simulink model "ExperimentalCarrier_longitudinal"  (R2015b)
settings: Solver=ode45  StartTime=0.0  StopTime=60  FixedStep=0.001  RelTol=1e-4
model workspace (MAT data in the model file):
  CX = [-0.020017155432; -0.0250180932111; -0.030544767781; -0.0366030177792; -0.0431954569041]
  CX_P = [-3.8788104025e-05; -0.000157009586721; -8.33005923499e-05; 4.36263205191e-05; 8.75463477638e-05]
  CX_Q = [-0.207993391526; -0.236116645752; -0.264091029583; -0.292079605385; -0.320346819683]
  CX_R = [0.00103448390012; 0.00120711118767; 0.00133502371584; 0.00146905219193; 0.0016515166303]
  CX_d = reshape([-0.0179596722301 -0.0197556406443 -0.0215296927775 -0.0233172355081 -0.0251411734088 0.00353274771863 0.00408472673345 0.00460460396215 0.00513024749002 0.00568462730478], [5 1 2])
  CX_d_elevator = [-0.0179596722301; -0.0197556406443; -0.0215296927775; -0.0233172355081; -0.0251411734088]
  CX_d_rudder = [0.00353274771863; 0.00408472673345; 0.00460460396215; 0.00513024749002; 0.00568462730478]
  CY = [-4.5217922426e-06; 5.22435851707e-05; 0.000183887113454; 0.000333475068731; 0.000452221434108]
  CY_P = [0.352257019544; 0.363263703068; 0.372310862359; 0.376200975649; 0.377300019734]
  CY_Q = [0.110043766373; 0.11079927373; 0.112561154643; 0.114510099317; 0.116086067683]
  CY_R = [-0.326040929997; -0.32773612119; -0.329287944874; -0.33055019267; -0.331668414023]
  CY_d = reshape([0.0148975523026 0.0150362935124 0.015237582339 0.0154527280836 0.0156448316098 -0.13717454765 -0.137491342129 -0.137816916372 -0.138147259306 -0.138463716116], [5 1 2])
  CY_d_elevator = [0.0148975523026; 0.0150362935124; 0.015237582339; 0.0154527280836; 0.0156448316098]
  CY_d_rudder = [-0.13717454765; -0.137491342129; -0.137816916372; -0.138147259306; -0.138463716116]
  CZ = [0.433918417301; 0.474298454266; 0.514671186482; 0.555148813041; 0.595722799276]
  CZ_P = [0.00129613826783; 0.00442759554205; 0.00267513559452; 0.000223228043457; -0.00031135300856]
  CZ_Q = [7.41020869928; 7.41837707941; 7.42599317709; 7.43441633219; 7.4434283008]
  CZ_R = [-0.030484458254; -0.0314562905176; -0.0323752658756; -0.0334837032738; -0.0349135867002]
  CZ_d = reshape([0.557451970659 0.557751465503 0.557962985265 0.558156625973 0.558318687373 -0.104459514841 -0.104809350426 -0.105143668837 -0.105483709566 -0.105819316132], [5 1 2])
  CZ_d_elevator = [0.557451970659; 0.557751465503; 0.557962985265; 0.558156625973; 0.558318687373]
  CZ_d_rudder = [-0.104459514841; -0.104809350426; -0.105143668837; -0.105483709566; -0.105819316132]
  Cl = [-1.35607961429e-06; -5.96188071166e-06; -1.67033646109e-05; -2.94231268293e-05; -4.01077970867e-05]
  Cl_P = [-0.439205034752; -0.440723709414; -0.442152638591; -0.443068299499; -0.443627112534]
  Cl_Q = [-0.00917034469699; -0.00927738512973; -0.00949166137223; -0.00975372945302; -0.0100173762744]
  Cl_R = [0.0707908045152; 0.0708836498468; 0.0709529443546; 0.0709782004888; 0.0709702581948]
  Cl_d = reshape([-0.00125631208593 -0.00127240477427 -0.00129594809443 -0.00132394457069 -0.00135365672185 0.0120340930302 0.0120431420253 0.0120538349209 0.012065931941 0.0120777084325], [5 1 2])
  Cl_d_elevator = [-0.00125631208593; -0.00127240477427; -0.00129594809443; -0.00132394457069; -0.00135365672185]
  Cl_d_rudder = [0.0120340930302; 0.0120431420253; 0.0120538349209; 0.012065931941; 0.0120777084325]
  Cm = [0.0125955960448; 0.00755459695358; 0.00246646731807; -0.00292807143153; -0.00862510234146]
  Cm_P = [-0.00284218408989; -0.0097092504066; -0.00585776139249; -0.000486652887433; 0.000677869990232]
  Cm_Q = [-9.33029736541; -9.33733537595; -9.34332688954; -9.35122395193; -9.36051345323]
  Cm_R = [0.0662348186498; 0.0683959531597; 0.0704584936088; 0.0729594772358; 0.0761904930638]
  Cm_d = reshape([-1.26929427701 -1.2696185084 -1.26973590838 -1.26980240453 -1.26978468603 0.228767161047 0.229455531687 0.230105888147 0.230769688943 0.231425434534], [5 1 2])
  Cm_d_elevator = [-1.26929427701; -1.2696185084; -1.26973590838; -1.26980240453; -1.26978468603]
  Cm_d_rudder = [0.228767161047; 0.229455531687; 0.230105888147; 0.230769688943; 0.231425434534]
  Cn = [-2.39196708194e-06; 2.19531005211e-05; 7.80516594694e-05; 0.000141460168108; 0.000191546816275]
  Cn_P = [-0.0138852805825; -0.0104525390167; -0.00804029890533; -0.00770122144879; -0.00830785414203]
  Cn_Q = [0.0468266728784; 0.0471357484906; 0.0478735856255; 0.0486865128781; 0.0493357339708]
  Cn_R = [-0.112685214148; -0.113184603314; -0.113623636715; -0.113957068484; -0.114242510185]
  Cn_d = reshape([0.00634316820633 0.00640010611535 0.00648337961591 0.00657205165139 0.00665055318483 -0.0584904156504 -0.058612540103 -0.0587418941859 -0.0588730038419 -0.0589956355318], [5 1 2])
  Cn_d_elevator = [0.00634316820633; 0.00640010611535; 0.00648337961591; 0.00657205165139; 0.00665055318483]
  Cn_d_rudder = [-0.0584904156504; -0.058612540103; -0.0587418941859; -0.0588730038419; -0.0589956355318]
  InertiaTensor = [1  0  0; 0  1  0; 0  0  1]
  alpha = [0.0698131700798; 0.0785398163397; 0.0872664625997; 0.0959931088597; 0.10471975512]
  alpha_ini = 0
  beta = 0
  centerOfGravity = -0.092
  estimatedVelocity = 14
  mass = 1.56
  mean_chord = 0.25
  q_ini = 0
  spanwidth = 1.5
  theta_ini = 0
undefined symbols (not defined in the file): Earth, m, s, U0, w0, WGS84
libraries: aerolibconvert2 x6, aerolibasang x2, aerolibfltsims x2, aerolib3dof2 x1, aerolibadyn x1, aerolibtransform2 x1, aerolibanimutils x1, aerolibatmos2 x1, aerolibgravity2 x1
settings Model: Creator=jruesch  LastModifiedBy=jruesch
settings DataIOCC: SaveFormat=Array
settings OptimizationCC: BlockReduction=off
settings HardwareCC: ProdBitPerPointer=32  ProdLargestAtomicFloat=None  ProdIntDivRoundTo=Undefined  ProdEndianess=Unspecified  ProdWordSize=32  ProdHWDeviceType=32-bit Generic
settings GRTTargetCC: GeneratePreprocessorConditionals=Disable all
settings ConfigComp: CovModelRefEnable=Off

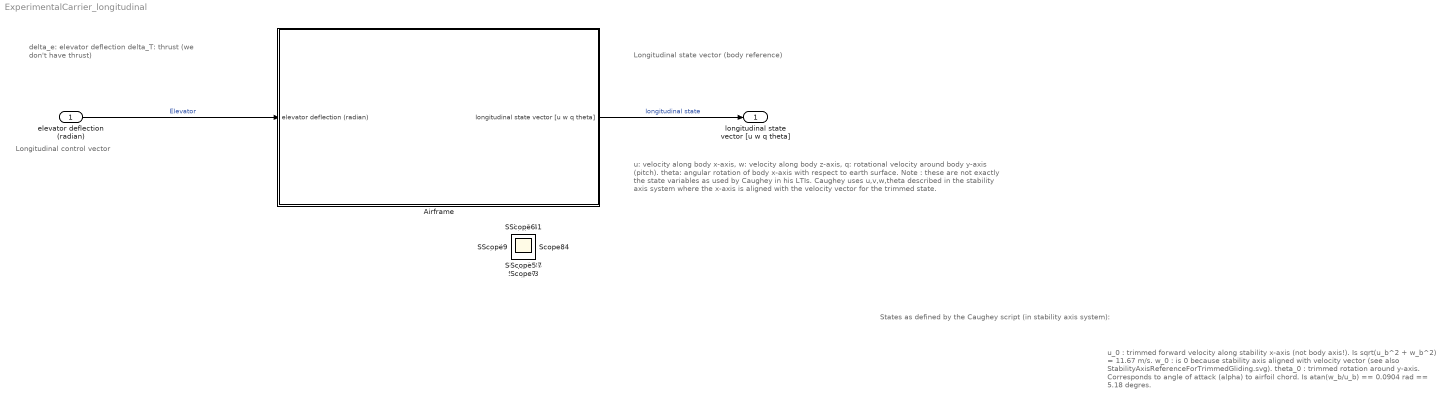
== system ExperimentalCarrier_longitudinal ==
  note: States as defined by the Caughey script (in stability axis system):
  note: u_0 : trimmed forward velocity along stability x-axis (not body axis!).
      | Is sqrt(u_b^2 + w_b^2) = 11.67 m/s.
      | w_0 : is 0 because stability axis aligned with velocity vector
      | (see also StabilityAxisReferenceForTrimmedGliding.svg).
      | theta_0 : trimmed rotation around y-axis. Corresponds
      | to angle of attack (alpha) to airfoil chord.
      | Is atan(w_b/u_b) == 0.0904 rad == 5.18 degres.
  note: delta_e: elevator deflection
      | delta_T: thrust (we don't have thrust)
  note: Longitudinal control vector
  note: u: velocity along body x-axis,
      | w: velocity along body z-axis,
      | q: rotational velocity around body y-axis (pitch).
      | theta: angular rotation of body x-axis with respect to earth surface.
      |
      | Note : these are not exactly the state variables as used by Caughey in his LTIs.
      | Caughey uses u,v,w,theta described in the stability axis system where the x-axis is aligned
      | with the velocity vector for the trimmed state.
  note: Longitudinal state vector (body reference)
  elevator deflection (radian) : Inport
  Airframe : Subsystem
      mask Display: image(imread('../../figures/Airframe.png'))
  longitudinal state vector [u w q theta] : Outport
  Scope{,1..41,43..45} (45 alike) : Scope
  wires:
  elevator deflection (radian)/1 -> Airframe/1(elevator deflection (radian))  "Elevator"
  Airframe/1(longitudinal state vector [u w q theta]) -> longitudinal state vector [u w q theta]/1  "longitudinal state"

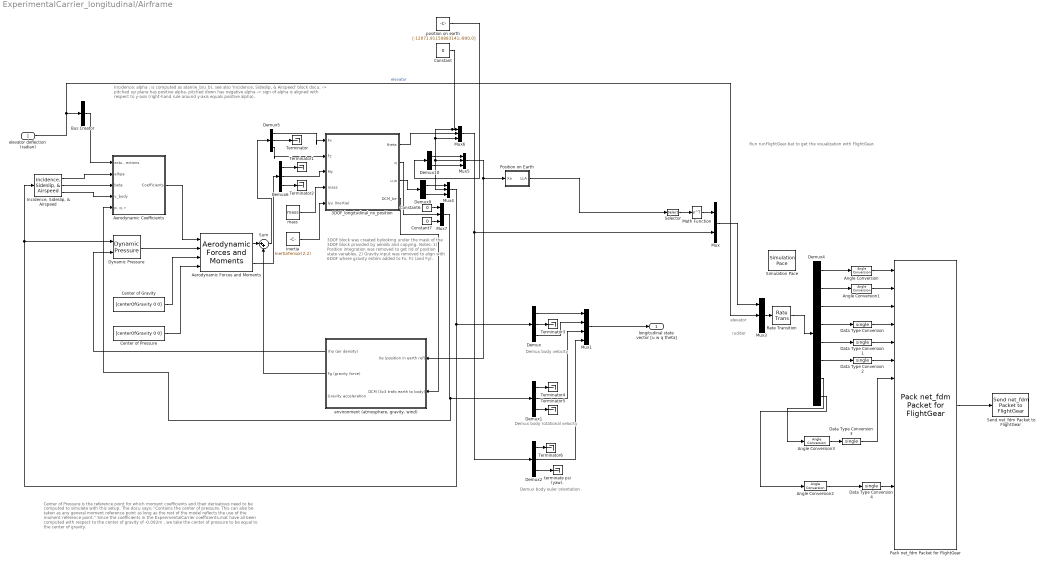
== system ExperimentalCarrier_longitudinal/Airframe ==
  note: 3DOF block was created bylooking under the mask of the 3DOF block provided by aerolib and copying.
      |
      | Notes:
      | 1) Position integration was removed to get rid of position state variables.
      | 2) Gravity input was removed to align with 6DOF where
      | gravity enters added to Fx, Fz (and Fy).
  note: rudder
  note: elevator
  note: Incidence:
      | alpha : is computed as atan(w_b/u_b), see also 'Incidence, Sideslip, & Airspeed' block docu.
      | -> pitched up plane has positive alpha, pitched down has negative alpha
      | -> sign of alpha is aligned with respect to y-axis (right-hand rule around y-axis equals positive alpha).
  note: Demux body velocity
  note: Run runFlightGear.bat to get the visualization with FlightGear.
  note: Center of Pressure is the reference point for which moment coefficients and their derivatives need to be computed to simulate with this setup.
      | The docu says: "Contains the center of pressure. This can also be taken as any general moment reference point as long as the rest of the model reflects the use of the moment reference point." Since the coefficients in the ExperimentalCarrier coefficients.mat have all been computed with respect to the center of gravity of -0.092m , we take the center of pressure to be equal to the center of gravity.
  note: Demux body rotational velocity
  note: Demux body euler orientation
  elevator deflection (radian) : Inport
  3DOF_longitudinal_no_position : Subsystem
  "Aerodynamic Forces and Moments " : aerolibadyn/Aerodynamic Forces and Moments   inputAxes=Body  outputForceAxes=Body  outputMomentAxes=Body  S=spanwidth*mean_chord  b=spanwidth  cbar=mean_chord
  Aerodynamic Coefficients : Subsystem
  Angle Conversion : aerolibconvert2/Angle Conversion  IU=deg  OU=rad
  Angle Conversion1 : aerolibconvert2/Angle Conversion  IU=deg  OU=rad
  Angle Conversion2 : aerolibconvert2/Angle Conversion  IU=rad  OU=deg
  Angle Conversion3 : aerolibconvert2/Angle Conversion  IU=rad  OU=deg
  Bus Creator : BusCreator  Inputs=1
  Center of Gravity : Constant  Value=[centerOfGravity 0 0]
  Center of Pressure : Constant  Value=[centerOfGravity 0 0]
  Constant : Constant  Value=0
  Constant6 : Constant  Value=0
  Constant7 : Constant  Value=0
  Data Type Conversion{,1..4} (5 alike) : DataTypeConversion  OutDataTypeStr=single
  Demux{,1..2,5..6} (5 alike) : Demux  Outputs=3
  Demux10 : Demux  Outputs=2
  Demux4 : Demux  Outputs=8
  Demux9 : Demux  Outputs=2
  Dynamic Pressure : aerolibasang/Dynamic Pressure
  "Incidence, Sideslip, & Airspeed" : aerolibasang/Incidence, Sideslip, & Airspeed
  Inertia : Constant  Value=InertiaTensor(2,2)
  Math Function : Math  Operator=transpose  SaturateOnIntegerOverflow=on
  Mux : Mux  Inputs=2
  Mux1 : Mux
  Mux{3..7} (5 alike) : Mux  Inputs=3
  Pack net_fdm Packet for FlightGear : aerolibfltsims/Pack net_fdm Packet for FlightGear  FlightGearVersion=v3.4  ShowPositionAttitudeInputs=on  ShowVelocityAccelerationInputs=off  ShowControlSurfacePositionInputs=on  ShowEngineFuelInputs=off  ShowLandingGearInputs=off  ShowEnvironmentInputs=off  SampleTime=1/30
  Position on Earth : Subsystem  Priority=1  TreatAsAtomicUnit=on
  Rate Transition : RateTransition  Integrity=off  OutPortSampleTime=1/30
  Selector : Selector  InputPortWidth=3  IndexOptions=Index vector (dialog)  Indices=[2 1 3]  OutputSizes=1
  Send net_fdm Packet to FlightGear : aerolibfltsims/Send net_fdm Packet to FlightGear  DestinationIpAddress=127.0.0.1  DestinationPort=5502  LocalIpPort=-1  varLen=off  SampleTime=1/30
  Simulation Pace : aerolibanimutils/Simulation Pace  SimulationPace=1  SleepMode=MATLAB Thread  OutputPaceError=off  SampleTime=1/30
      settings: AttributesFormatString=%<SimulationPace> sec/sec
  Sum : Sum  Inputs=|++
  Terminator{,1..6} (7 alike) : Terminator
  "environment (atmosphere, gravity, wind)" : Subsystem
  mass : Constant  Value=mass
  position on earth : Constant  Value=[-12071.91150883141;-800.0]
  terminate psi (yaw). : Terminator
  longitudinal state vector [u w q theta] : Outport
  wires:
  "Aerodynamic Forces and Moments "/1 -> Sum/1
  "Aerodynamic Forces and Moments "/2 -> Demux6/1
  Center of Gravity/1 -> "Aerodynamic Forces and Moments "/3
  Center of Pressure/1 -> "Aerodynamic Forces and Moments "/4
  Dynamic Pressure/1 -> "Aerodynamic Forces and Moments "/2
  Position on Earth/1(LLA) -> Selector/1
  Math Function/1 -> Mux/1
  Mux/1 -> Mux3/1
  Selector/1 -> Math Function/1
  "environment (atmosphere, gravity, wind)"/1(rho (air density)) -> Dynamic Pressure/2
  "Incidence, Sideslip, & Airspeed"/1 -> Aerodynamic Coefficients/2(alhpa)
  "Incidence, Sideslip, & Airspeed"/2 -> Aerodynamic Coefficients/3(beta)
  "Incidence, Sideslip, & Airspeed"/3 -> Aerodynamic Coefficients/4(v_body)
  Aerodynamic Coefficients/1(Coefficients) -> "Aerodynamic Forces and Moments "/1
  Bus Creator/1 -> Aerodynamic Coefficients/1(actuator deflections)
  elevator deflection (radian)/1 -> Mux3/2, Bus Creator/1  "elevator"
  Demux/1 -> Mux1/1
  Demux/3 -> Mux1/2
  Demux1/2 -> Mux1/3
  Demux2/2 -> Mux1/4
  Demux2/3 -> terminate psi (yaw)./1
  Mux1/1 -> longitudinal state vector [u w q theta]/1
  Pack net_fdm Packet for FlightGear/1 -> Send net_fdm Packet to FlightGear/1
  Demux4/1 -> Angle Conversion/1
  Demux4/2 -> Angle Conversion1/1
  Demux4/3 -> Pack net_fdm Packet for FlightGear/3
  Demux4/4 -> Data Type Conversion/1
  Demux4/5 -> Data Type Conversion1/1
  Demux4/6 -> Data Type Conversion2/1
  Rate Transition/1 -> Demux4/1
  Angle Conversion/1 -> Pack net_fdm Packet for FlightGear/1
  Angle Conversion1/1 -> Pack net_fdm Packet for FlightGear/2
  Data Type Conversion/1 -> Pack net_fdm Packet for FlightGear/4
  Data Type Conversion1/1 -> Pack net_fdm Packet for FlightGear/5
  Data Type Conversion2/1 -> Pack net_fdm Packet for FlightGear/6
  Mux3/1 -> Rate Transition/1
  Demux4/7 -> Angle Conversion3/1
  Demux4/8 -> Angle Conversion2/1
  Data Type Conversion3/1 -> Pack net_fdm Packet for FlightGear/7
  Data Type Conversion4/1 -> Pack net_fdm Packet for FlightGear/13
  Angle Conversion2/1 -> Data Type Conversion4/1
  Angle Conversion3/1 -> Data Type Conversion3/1
  3DOF_longitudinal_no_position/3("u,w  ") -> Demux9/1
  Demux5/1 -> 3DOF_longitudinal_no_position/1(Fx)
  Demux5/3 -> 3DOF_longitudinal_no_position/2(Fz)
  Demux5/2 -> Terminator/1
  Demux6/1 -> Terminator1/1
  Demux6/3 -> Terminator2/1
  Demux6/2 -> 3DOF_longitudinal_no_position/3(My)
  Demux9/1 -> Mux4/1
  Demux9/2 -> Mux4/3
  Mux4/1 -> Demux/1, "Incidence, Sideslip, & Airspeed"/1, Dynamic Pressure/1
  Constant/1 -> Mux6/3, Mux5/2, Mux4/2, Mux6/1
  position on earth/1 -> Demux10/1
  Demux10/2 -> Mux5/3
  Demux10/1 -> Mux5/1
  Mux5/1 -> "environment (atmosphere, gravity, wind)"/1(Xe (position in earth ref)), Position on Earth/1(Xe)
  3DOF_longitudinal_no_position/1(theta) -> Mux6/2
  Mux6/1 -> Mux/2, Demux2/1
  "environment (atmosphere, gravity, wind)"/2(Fg (gravity force)) -> Sum/2
  3DOF_longitudinal_no_position/4(DCM_be) -> "environment (atmosphere, gravity, wind)"/2(DCM (3x3 trafo earth to body))
  Constant6/1 -> Mux7/1
  Constant7/1 -> Mux7/3
  3DOF_longitudinal_no_position/2("q ") -> Mux7/2
  Mux7/1 -> Aerodynamic Coefficients/5("p, q, r"), Demux1/1
  Demux/2 -> Terminator3/1
  Demux1/1 -> Terminator4/1
  Demux1/3 -> Terminator5/1
  Demux2/1 -> Terminator6/1
  mass/1 -> 3DOF_longitudinal_no_position/4(mass)
  Inertia/1 -> 3DOF_longitudinal_no_position/5(Iyy (Inertia))
  Sum/1 -> Demux5/1

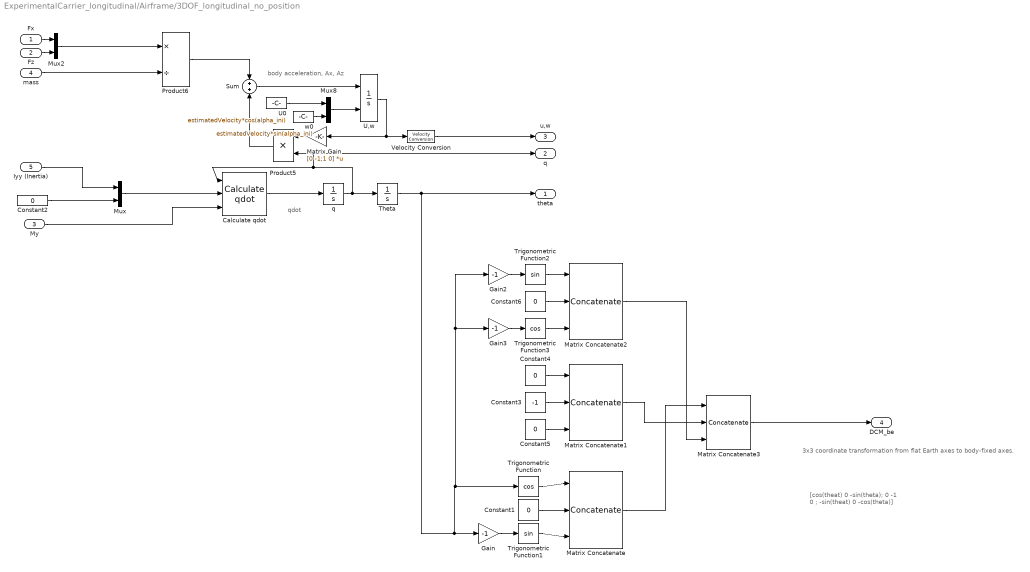
== system ExperimentalCarrier_longitudinal/Airframe/3DOF_longitudinal_no_position ==
  note: qdot
  note: body acceleration, Ax, Az
  note: 3x3 coordinate transformation from flat Earth axes to body-fixed axes.
  note: [cos(theat) 0 -sin(theta);
      |  0              -1 0            ;
      |  -sin(theat) 0 -cos(theta)]
  Fx : Inport
  Fz : Inport  Port=2
  My : Inport  Port=3
  mass : Inport  Port=4
  Iyy (Inertia) : Inport  Port=5
  Calculate qdot : aerolib3dof2/3DOF (Body Axes)/Calculate qdot
  Constant{1,4..6} (4 alike) : Constant  Value=0
  Constant2 : Constant  Value=0  OutDataTypeStr=Inherit: Inherit via back propagation
  Constant3 : Constant  Value=-1
  Gain : Gain  Gain=-1
  Gain2 : Gain  Gain=-1
  Gain3 : Gain  Gain=-1
  Matrix Concatenate : Concatenate  NumInputs=3  ConcatenateDimension=2
  Matrix Concatenate1 : Concatenate  NumInputs=3  ConcatenateDimension=2
  Matrix Concatenate2 : Concatenate  NumInputs=3  ConcatenateDimension=2
  Matrix Concatenate3 : Concatenate  NumInputs=3  Mode=Multidimensional array  ConcatenateDimension=2
  Matrix Gain : Gain  Gain=[0 -1;1 0]  Multiplication=Matrix(K*u)  SaturateOnIntegerOverflow=on  OutDataTypeStr=Inherit: Same as input  ParamDataTypeStr=Inherit: Same as input
  Mux : Mux  Inputs=2
  Mux2 : Mux  Inputs=2
  Mux8 : Mux  Inputs=2
  Product5 : Product  SaturateOnIntegerOverflow=on  InputSameDT=on  OutDataTypeStr=Inherit: Same as first input
  Product6 : Product  Inputs=*/  SaturateOnIntegerOverflow=on  OutDataTypeStr=Inherit: Same as first input
  Sum : Sum  SaturateOnIntegerOverflow=on
  Theta : Integrator  InitialCondition=theta_ini
  Trigonometric Function : Trigonometry  Operator=cos
  Trigonometric Function1 : Trigonometry
  Trigonometric Function2 : Trigonometry
  Trigonometric Function3 : Trigonometry  Operator=cos
  U,w : Integrator  InitialConditionSource=external  InitialCondition=convvel([U0 w0],'m/s','m/s')
  U0 : Constant  Value=estimatedVelocity*cos(alpha_ini)
  Velocity Conversion : aerolibconvert2/Velocity Conversion  IU=m/s  OU=m/s
  q : Integrator  InitialCondition=q_ini
  w0 : Constant  Value=estimatedVelocity*sin(alpha_ini)
  theta : Outport  InitialOutput=0
  "q " : Outport  Port=2  InitialOutput=0
  "u,w  " : Outport  Port=3  InitialOutput=0
  DCM_be : Outport  Port=4
  wires:
  Fz/1 -> Mux2/2
  Product6/1 -> Sum/1
  Mux8/1 -> U,w/2
  My/1 -> Calculate qdot/3
  Fx/1 -> Mux2/1
  U0/1 -> Mux8/1
  mass/1 -> Product6/2
  U,w/1 -> Matrix Gain/1, Velocity Conversion/1
  w0/1 -> Mux8/2
  Sum/1 -> U,w/1
  q/1 -> Calculate qdot/1, "q "/1, Product5/2, Theta/1
  Matrix Gain/1 -> Product5/1
  Velocity Conversion/1 -> "u,w  "/1
  Calculate qdot/1 -> q/1
  Product5/1 -> Sum/2
  Mux2/1 -> Product6/1
  Constant2/1 -> Mux/2
  Mux/1 -> Calculate qdot/2
  Iyy (Inertia)/1 -> Mux/1
  Theta/1 -> theta/1, Gain/1, Gain3/1, Gain2/1, Trigonometric Function/1
  Trigonometric Function/1 -> Matrix Concatenate/1
  Gain/1 -> Trigonometric Function1/1
  Trigonometric Function1/1 -> Matrix Concatenate/3
  Constant1/1 -> Matrix Concatenate/2
  Constant3/1 -> Matrix Concatenate1/2
  Constant4/1 -> Matrix Concatenate1/1
  Constant5/1 -> Matrix Concatenate1/3
  Trigonometric Function2/1 -> Matrix Concatenate2/1
  Gain2/1 -> Trigonometric Function2/1
  Trigonometric Function3/1 -> Matrix Concatenate2/3
  Gain3/1 -> Trigonometric Function3/1
  Constant6/1 -> Matrix Concatenate2/2
  Matrix Concatenate/1 -> Matrix Concatenate3/1
  Matrix Concatenate1/1 -> Matrix Concatenate3/2
  Matrix Concatenate2/1 -> Matrix Concatenate3/3
  Matrix Concatenate3/1 -> DCM_be/1

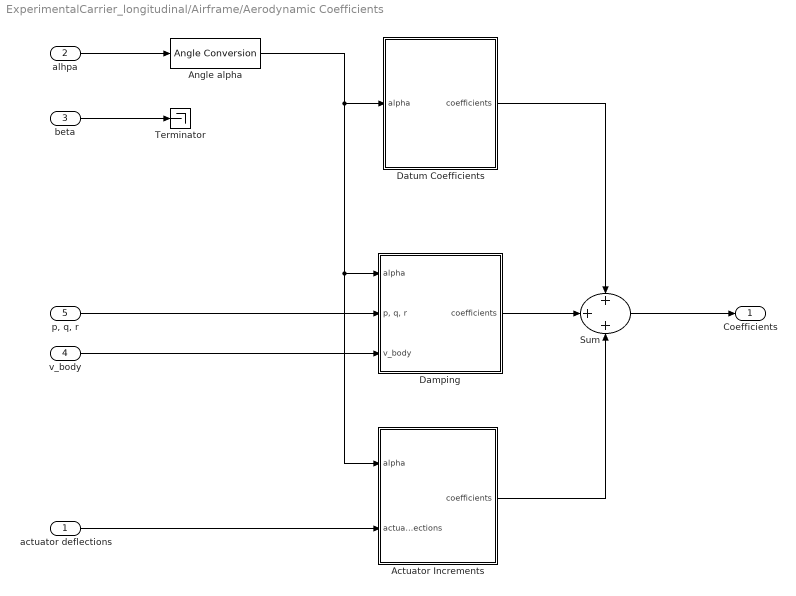
== system ExperimentalCarrier_longitudinal/Airframe/Aerodynamic Coefficients ==
  actuator deflections : Inport
  alhpa : Inport  Port=2
  beta : Inport  Port=3
  v_body : Inport  Port=4
  "p, q, r" : Inport  Port=5
  Actuator Increments : Subsystem
  Angle alpha : aerolibconvert2/Angle Conversion  IU=rad  OU=deg
  Damping : Subsystem
  Datum Coefficients : Subsystem
  Sum : Sum  Inputs=+++
  Terminator : Terminator
  Coefficients : Outport
  wires:
  alhpa/1 -> Angle alpha/1
  Angle alpha/1 -> Actuator Increments/1(alpha), Damping/1(alpha), Datum Coefficients/1(alpha)
  Datum Coefficients/1(coefficients) -> Sum/1
  "p, q, r"/1 -> Damping/2("p, q, r")
  Damping/1(coefficients) -> Sum/2
  Sum/1 -> Coefficients/1
  v_body/1 -> Damping/3(v_body)
  beta/1 -> Terminator/1
  actuator deflections/1 -> Actuator Increments/2(actuator deflections)
  Actuator Increments/1(coefficients) -> Sum/3

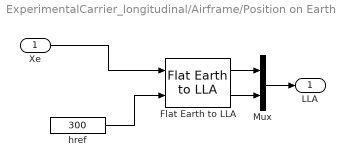
== system ExperimentalCarrier_longitudinal/Airframe/Position on Earth ==
  Xe : Inport
  Flat Earth to LLA : aerolibtransform2/Flat Earth to LLA  units=Metric (MKS)  ptype=Earth (WGS84)  F=1/298.257223563  R=6378137  LL0=[37.628738616666666,-1.223933911333333e+02]  psi=0
  Mux : Mux  Inputs=2
  href : Constant  Value=300
  LLA : Outport
  wires:
  Mux/1 -> LLA/1
  Xe/1 -> Flat Earth to LLA/1
  Flat Earth to LLA/1 -> Mux/1
  Flat Earth to LLA/2 -> Mux/2
  href/1 -> Flat Earth to LLA/2

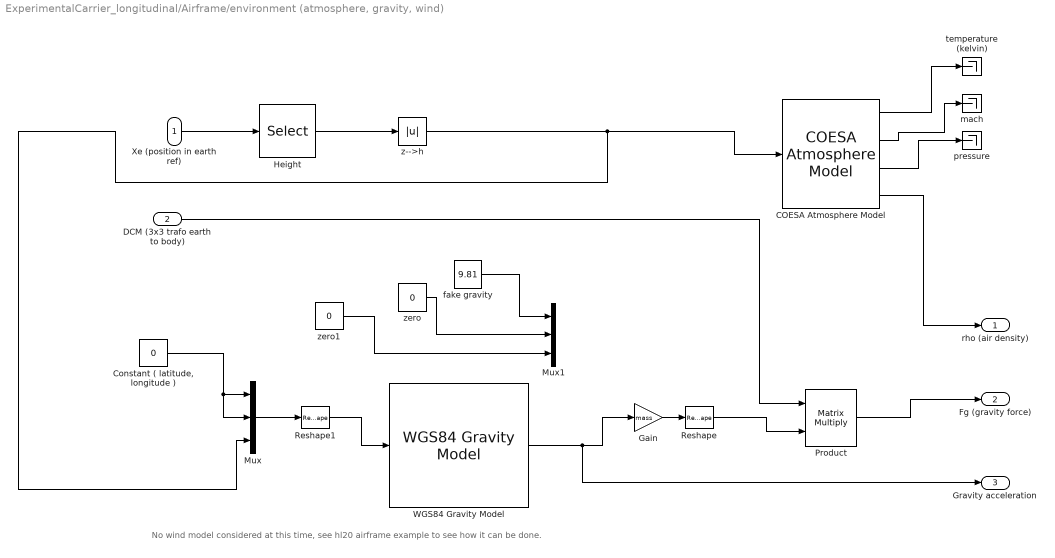
== system ExperimentalCarrier_longitudinal/Airframe/environment (atmosphere, gravity, wind) ==
  note: No wind model considered at this time, see hl20 airframe example to see how it can be done.
  Xe (position in earth ref) : Inport
  DCM (3x3 trafo earth to body) : Inport  Port=2
  COESA Atmosphere Model : aerolibatmos2/COESA Atmosphere Model  units=Metric (MKS)  spec=1976 COESA-extended U.S. Standard Atmosphere  model=Profile  profile_var=High temperature  profile_percent=1%  profile_alt=5 km (16404 ft)  envelope_var=High temperature  envelope_percent=1%  action=Warning
  "Constant ( latitude, longitude )" : Constant  Value=0
  Gain : Gain  Gain=mass
  Height : Selector  InputPortWidth=3  IndexOptions=Index vector (dialog)  Indices=[3]  OutputSizes=1
  Mux : Mux  Inputs=3
  Mux1 : Mux  Inputs=3
  Product : Product  Multiplication=Matrix(*)
  Reshape : Reshape
  Reshape1 : Reshape
  "WGS84 Gravity Model " : aerolibgravity2/WGS84 Gravity Model   model=WGS84 Taylor Series  units=Metric (MKS)  no_atmos=on  precessing=on  jd_loc=off  month=October  day=10  year=2004  no_centrifugal=on  action=Warning
  fake gravity : Constant  Value=9.81
  mach : Terminator
  pressure : Terminator
  temperature (kelvin) : Terminator
  z-->h : Abs  SaturateOnIntegerOverflow=on
  zero : Constant  Value=0
  zero1 : Constant  Value=0
  rho (air density) : Outport
  Fg (gravity force) : Outport  Port=2
  Gravity acceleration : Outport  Port=3
  wires:
  Xe (position in earth ref)/1 -> Height/1
  Height/1 -> z-->h/1
  z-->h/1 -> Mux/3, COESA Atmosphere Model/1
  COESA Atmosphere Model/4 -> rho (air density)/1
  COESA Atmosphere Model/1 -> temperature (kelvin)/1
  COESA Atmosphere Model/2 -> mach/1
  COESA Atmosphere Model/3 -> pressure/1
  "Constant ( latitude, longitude )"/1 -> Mux/1, Mux/2
  Mux/1 -> Reshape1/1
  fake gravity/1 -> Mux1/1
  Gain/1 -> Reshape/1
  Reshape/1 -> Product/2
  DCM (3x3 trafo earth to body)/1 -> Product/1
  Product/1 -> Fg (gravity force)/1
  zero/1 -> Mux1/2
  zero1/1 -> Mux1/3
  Reshape1/1 -> "WGS84 Gravity Model "/1
  "WGS84 Gravity Model "/1 -> Gravity acceleration/1, Gain/1

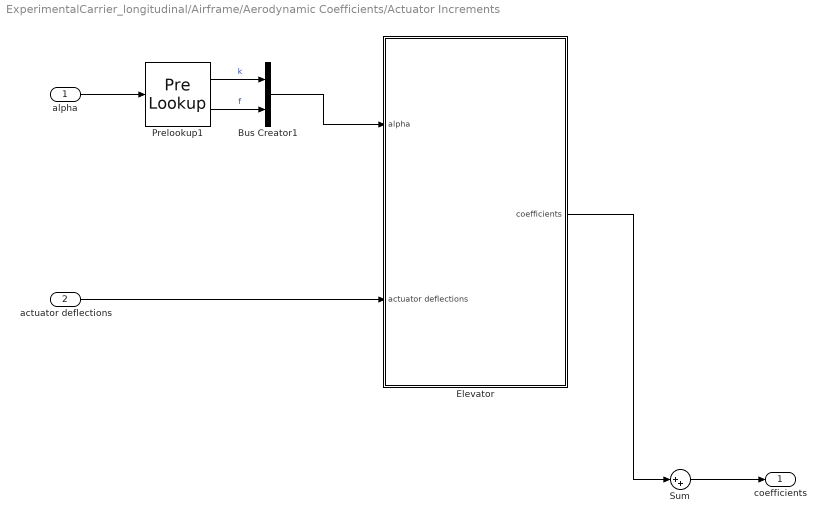
== system ExperimentalCarrier_longitudinal/Airframe/Aerodynamic Coefficients/Actuator Increments ==
  alpha : Inport
  actuator deflections : Inport  Port=2
  Bus Creator1 : BusCreator  Inputs=2
  Elevator : Subsystem
  Prelookup1 : PreLookup  BreakpointsData=alpha*180/pi  ExtrapMethod=Linear
  Sum : Sum  Inputs=|++
  coefficients : Outport
  wires:
  alpha/1 -> Prelookup1/1
  actuator deflections/1 -> Elevator/2(actuator deflections)
  Elevator/1(coefficients) -> Sum/1
  Sum/1 -> coefficients/1
  Prelookup1/1 -> Bus Creator1/1  "k"
  Prelookup1/2 -> Bus Creator1/2  "f"
  Bus Creator1/1 -> Elevator/1(alpha)

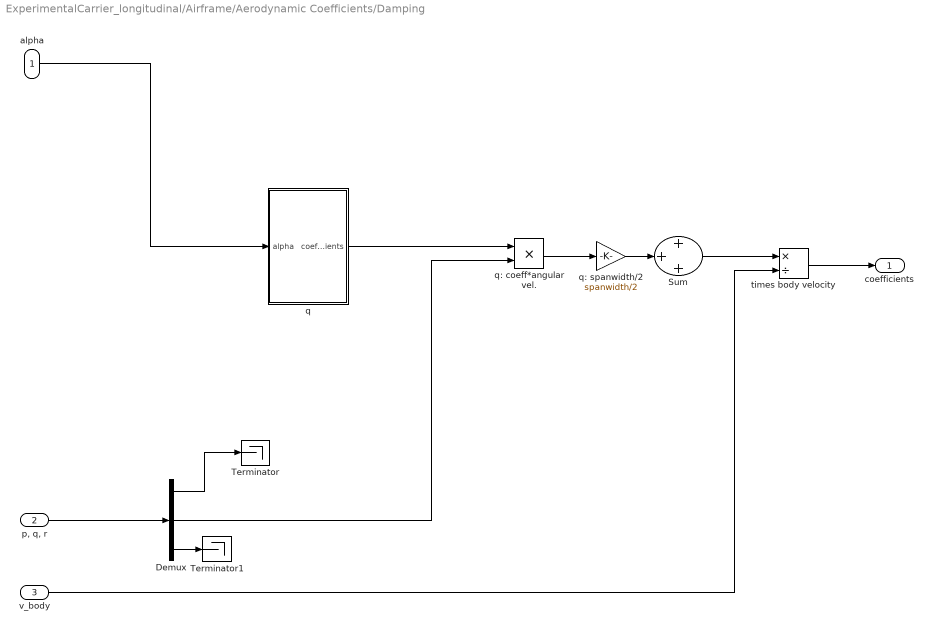
== system ExperimentalCarrier_longitudinal/Airframe/Aerodynamic Coefficients/Damping ==
  alpha : Inport
  "p, q, r" : Inport  Port=2
  v_body : Inport  Port=3
  Demux : Demux  Outputs=3
  Sum : Sum  Inputs=+++
  Terminator : Terminator
  Terminator1 : Terminator
  q : Subsystem
  q: coeff*angular vel. : Product
  q: spanwidth/2 : Gain  Gain=spanwidth/2
  times body velocity : Product  Inputs=*/
  coefficients : Outport
  wires:
  alpha/1 -> q/1(alpha)
  "p, q, r"/1 -> Demux/1
  Sum/1 -> times body velocity/1
  v_body/1 -> times body velocity/2
  q/1(coefficients) -> q: coeff*angular vel./1
  q: spanwidth/2/1 -> Sum/2
  q: coeff*angular vel./1 -> q: spanwidth/2/1
  Demux/2 -> q: coeff*angular vel./2
  times body velocity/1 -> coefficients/1
  Demux/1 -> Terminator/1
  Demux/3 -> Terminator1/1

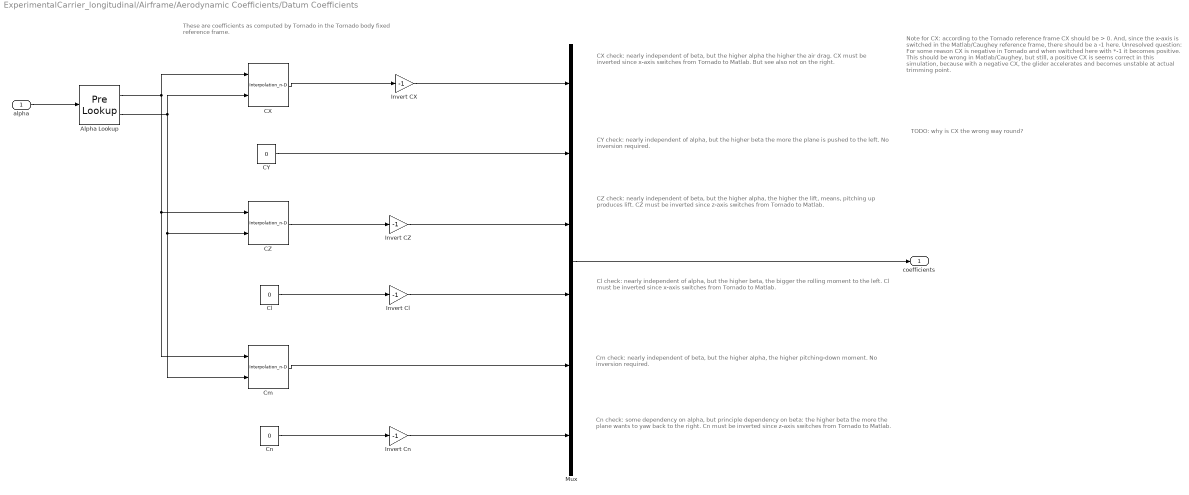
== system ExperimentalCarrier_longitudinal/Airframe/Aerodynamic Coefficients/Datum Coefficients ==
  note: Cl check: nearly independent of alpha, but the higher beta, the bigger the rolling moment to the left. Cl must be inverted since x-axis switches from Tornado to Matlab.
  note: CY check: nearly independent of alpha, but
      | the higher beta the more the plane is pushed to the left. No inversion required.
  note: These are coefficients as computed by Tornado in the
      | Tornado body fixed reference frame.
  note: Cm check: nearly independent of beta, but the higher alpha, the higher pitching-down moment. No inversion required.
  note: CZ check: nearly independent of beta, but the higher alpha, the higher the lift, means, pitching up produces lift. CZ must be inverted since z-axis switches from Tornado to Matlab.
  note: Note for CX: according to the Tornado reference frame
      | CX should be > 0. And, since the x-axis is switched in the
      | Matlab/Caughey reference frame, there should be a -1 here.
      | Unresolved question: For some reason CX is negative in Tornado
      | and when switched here with *-1 it becomes positive. This should
      | be wrong in Matlab/Caughey, but still, a positive CX is seems correct
      | in this simulation, because with a negative CX, the glider
      | accelerates and becomes unstable at actual trimming point.
  note: Cn check: some dependency on alpha, but principle dependency on beta: the higher beta the more the plane wants to yaw back to the right. Cn must be inverted since z-axis switches from Tornado to Matlab.
  note: CX check: nearly independent of beta, but the higher alpha the higher the air drag. CX must be inverted since x-axis switches from Tornado to Matlab. But see also not on the right.
  note: TODO:
      | why is CX the wrong way round?
  alpha : Inport
  Alpha Lookup : PreLookup  BreakpointsData=alpha*180/pi  ExtrapMethod=Linear
  CX : Interpolation_n-D  NumberOfTableDimensions=1  Table=CX  InternalRulePriority=Speed
      settings: InputPortMap=u0,u1
  CY : Constant  Value=0
  CZ : Interpolation_n-D  NumberOfTableDimensions=1  Table=CZ  InternalRulePriority=Speed
      settings: InputPortMap=u0,u1
  Cl : Constant  Value=0
  Cm : Interpolation_n-D  NumberOfTableDimensions=1  Table=Cm  InternalRulePriority=Speed
      settings: InputPortMap=u0,u1
  Cn : Constant  Value=0
  Invert CX : Gain  Gain=-1
  Invert CZ : Gain  Gain=-1
  Invert Cl : Gain  Gain=-1
  Invert Cn : Gain  Gain=-1
  Mux : Mux  Inputs=6
  coefficients : Outport
  wires:
  Alpha Lookup/1 -> Cm/1, CZ/1, CX/1
  Alpha Lookup/2 -> Cm/2, CZ/2, CX/2
  alpha/1 -> Alpha Lookup/1
  Mux/1 -> coefficients/1
  CZ/1 -> Invert CZ/1
  CY/1 -> Mux/2
  CX/1 -> Invert CX/1
  Cl/1 -> Invert Cl/1
  Cn/1 -> Invert Cn/1
  Invert CZ/1 -> Mux/3
  Invert Cl/1 -> Mux/4
  Invert Cn/1 -> Mux/6
  Invert CX/1 -> Mux/1
  Cm/1 -> Mux/5

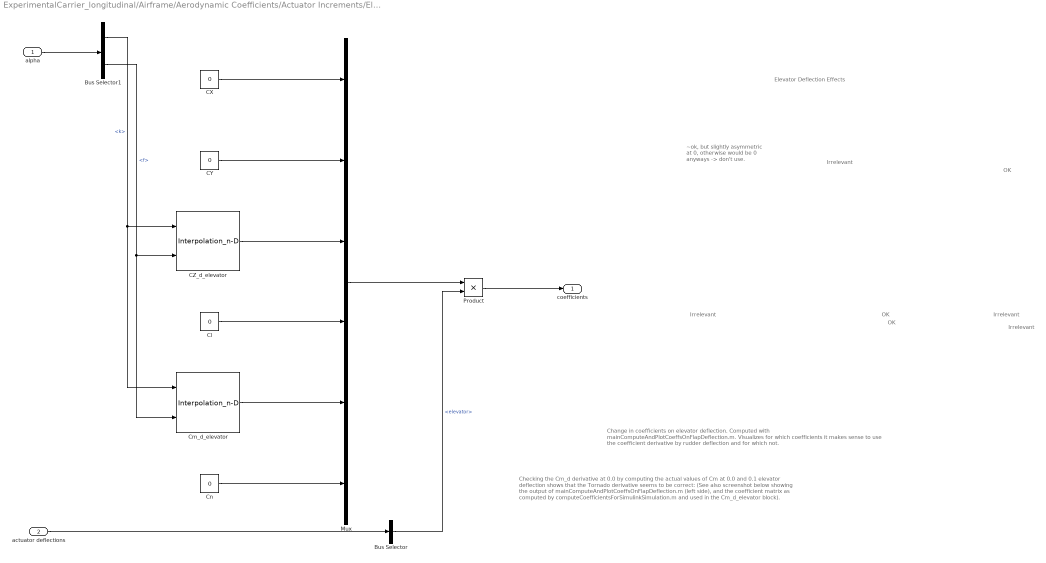
== system ExperimentalCarrier_longitudinal/Airframe/Aerodynamic Coefficients/Actuator Increments/Elevator ==
  note: Checking the Cm_d derivative at 0.0 by computing the actual values of Cm at 0.0 and 0.1 elevator deflection shows that the Tornado derivative seems to be correct:
      | (See also screenshot below showing the output of mainComputeAndPlotCoeffsOnFlapDeflection.m (left side), and the coefficient matrix as computed by computeCoefficientsForSimulinkSimulation.m and used in the Cm_d_elevator block).
  note: OK
  note: Irrelevant
  note: ~ok, but slightly
      | asymmetric at 0,
      | otherwise would
      | be 0 anyways
      | -> don't use.
  note: Irrelevant
  note: OK
  note: Irrelevant
  note: Change in coefficients on elevator deflection. Computed with mainComputeAndPlotCoeffsOnFlapDeflection.m.
      | Visualizes for which coefficients it makes sense to use the coefficient derivative by rudder deflection and for which not.
  note: Elevator Deflection Effects
  note: OK
  note: Irrelevant
  alpha : Inport
  actuator deflections : Inport  Port=2
  Bus Selector : BusSelector  OutputSignals=elevator
  Bus Selector1 : BusSelector  OutputSignals=k,f
  CX : Constant  Value=0
  CY : Constant  Value=0
  CZ_d_elevator : Interpolation_n-D  NumberOfTableDimensions=1  Table=CZ_d_elevator  InternalRulePriority=Speed
      settings: InputPortMap=u0,u1
  Cl : Constant  Value=0
  Cm_d_elevator : Interpolation_n-D  NumberOfTableDimensions=1  Table=Cm_d_elevator  InternalRulePriority=Speed
      settings: InputPortMap=u0,u1
  Cn : Constant  Value=0
  Mux : Mux  Inputs=6
  Product : Product
  coefficients : Outport
  wires:
  Bus Selector1/1 -> Cm_d_elevator/1, CZ_d_elevator/1  "<k>"
  Bus Selector1/2 -> Cm_d_elevator/2, CZ_d_elevator/2  "<f>"
  alpha/1 -> Bus Selector1/1
  CY/1 -> Mux/2
  CZ_d_elevator/1 -> Mux/3
  Cm_d_elevator/1 -> Mux/5
  actuator deflections/1 -> Bus Selector/1
  Product/1 -> coefficients/1
  Bus Selector/1 -> Product/2  "<elevator>"
  Mux/1 -> Product/1
  Cl/1 -> Mux/4
  Cn/1 -> Mux/6
  CX/1 -> Mux/1

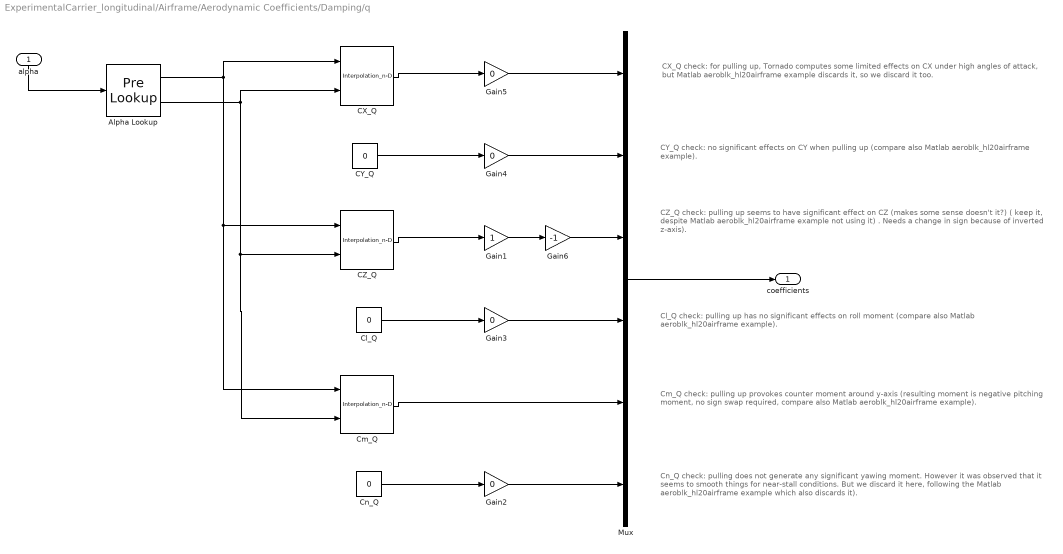
== system ExperimentalCarrier_longitudinal/Airframe/Aerodynamic Coefficients/Damping/q ==
  note: CX_Q check: for pulling up, Tornado computes some limited effects on CX under high angles of attack, but Matlab aeroblk_hl20airframe example discards it, so we discard it too.
  note: CZ_Q check: pulling up seems to have significant effect on CZ (makes some sense doesn't it?) ( keep it, despite Matlab aeroblk_hl20airframe example not using it) . Needs a change in sign because of inverted z-axis).
  note: Cl_Q check: pulling up has no significant effects on roll moment (compare also Matlab aeroblk_hl20airframe example).
  note: Cn_Q check: pulling does not generate any significant yawing moment. However it was observed that it seems to smooth things for near-stall conditions. But we discard it here, following the Matlab aeroblk_hl20airframe example which also discards it).
  note: Cm_Q check: pulling up provokes counter moment around y-axis (resulting moment is negative pitching moment, no sign swap required, compare also Matlab aeroblk_hl20airframe example).
  note: CY_Q check: no significant effects on CY when pulling up (compare also Matlab aeroblk_hl20airframe example).
  alpha : Inport
  Alpha Lookup : PreLookup  BreakpointsData=alpha*180/pi  ExtrapMethod=Linear
  CX_Q : Interpolation_n-D  NumberOfTableDimensions=1  Table=CX_Q  InternalRulePriority=Speed
      settings: InputPortMap=u0,u1
  CY_Q : Constant  Value=0
  CZ_Q : Interpolation_n-D  NumberOfTableDimensions=1  Table=CZ_Q  InternalRulePriority=Speed
      settings: InputPortMap=u0,u1
  Cl_Q : Constant  Value=0
  Cm_Q : Interpolation_n-D  NumberOfTableDimensions=1  Table=Cm_Q  InternalRulePriority=Speed
      settings: InputPortMap=u0,u1
  Cn_Q : Constant  Value=0
  Gain1 : Gain
  Gain{2..5} (4 alike) : Gain  Gain=0
  Gain6 : Gain  Gain=-1
  Mux : Mux  Inputs=6
  coefficients : Outport
  wires:
  CZ_Q/1 -> Gain1/1
  Alpha Lookup/2 -> CZ_Q/2, Cm_Q/2, CX_Q/2
  CY_Q/1 -> Gain4/1
  Alpha Lookup/1 -> CZ_Q/1, Cm_Q/1, CX_Q/1
  Cm_Q/1 -> Mux/5
  Mux/1 -> coefficients/1
  alpha/1 -> Alpha Lookup/1
  CX_Q/1 -> Gain5/1
  Gain1/1 -> Gain6/1
  Cn_Q/1 -> Gain2/1
  Gain2/1 -> Mux/6
  Cl_Q/1 -> Gain3/1
  Gain3/1 -> Mux/4
  Gain4/1 -> Mux/2
  Gain5/1 -> Mux/1
  Gain6/1 -> Mux/3
